simulink model "Samuno_Experimental_2024b"  (R2024b)
settings: Solver=ode4  StartTime=0.0  StopTime=Dur  FixedStep=simulation_ts  RelTol=1e-3  AbsTol=1e-3
InitFcn:
  | run("init_parts.m");
model workspace (MAT data in the model file):
  Control_Range_Lim = 0.2086
  D_Heading = 0
  I_Heading = 0
  P_Heading = 1
  control_ts = 0.4
  kd_pitch = 0
  kd_roll = 0.1
  kp_pitch = 4
  kp_roll = 4
  random_velocity = 0.72
  switch_val = 0.1032
values from neighbouring files (symbols this model uses):
  Force_Scale = 1    [init_parts.m]
  gravity = 9.81    [init_parts.m]
  m = (4*pi*rho*a*b*b)/3    (= 4.90497489324)    [init_parts.m]
  noise_mean = 1    [init_parts.m]
  noise_sample_time = 0.001    [init_parts.m]
  noise_var = 0.001    [init_parts.m]
  Nose = evalin('base', 'Nose')    [createSimulinkGUI_2024b.m]
  xCOB = xSliderCOB.Value    [createSimulinkGUI_2024b.m]    (also in init_parts.m = 0)
  zCOB = ySliderCOB.Value    [createSimulinkGUI_2024b.m]    (also in init_parts.m = 0)
undefined symbols (not defined in the file or in its folder): Caudal, colors, Mid_Body, Mid_Fins, Pect, Pedunc, X, Y, Z
libraries: nesl_utility x92, sm_lib x60
(part 3 of 3)

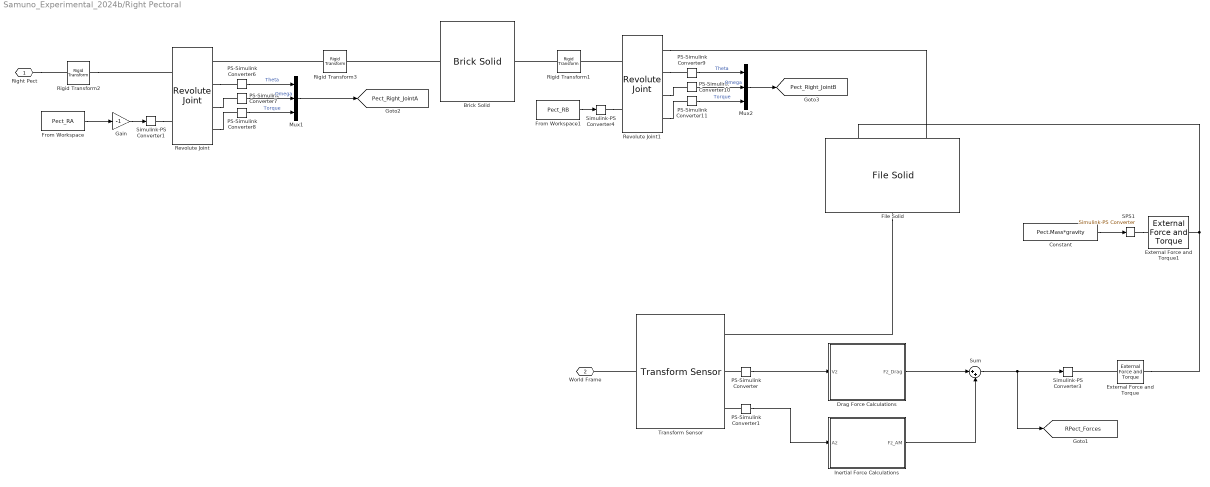
== system Samuno_Experimental_2024b/Right Pectoral ==
  Brick Solid : sm_lib/Body Elements/Brick Solid  BrickDimensions=[.01 .001 .001]  BrickDimensionsUnits=m  ExportEntireGeometry=off  InertiaType=CalculateFromGeometry  BasedOnType=Mass  Density=1000  DensityUnits=kg/m^3  Mass=0  MassUnits=kg  CenterOfMass=[0 0 0]  CenterOfMassUnits=m  MomentsOfInertia=[1 1 1]  MomentsOfInertiaUnits=kg*m^2  ProductsOfInertia=[0 0 0]  ProductsOfInertiaUnits=kg*m^2  GraphicType=FromGeometry  MarkerShape=Sphere  MarkerSize=10  GraphicVisPropType=SimpleVisualProperties  GraphicDiffuseColor=[0.5 0.5 0.5]  GraphicOpacity=1  GraphicSpecularColor=[0.5 0.5 0.5 1.0]  GraphicAmbientColor=[0.15 0.15 0.15 1.0]  GraphicEmissiveColor=[0.0 0.0 0.0 1.0]  GraphicShininess=75  DoExposeReferenceFrame=on  SerializedFrames=<Frames><Frame><Id>Frame1</Id><Value><Name>F1</Name><Origin><Source>ReferenceFrame</Source><FeatureName></FeatureName></Origin><PrimaryAxis><DefinedDirection>+Y</DefinedDirection><Source>GeometricFeature</Source><SourceDirection>+Z</SourceDirection><FeatureName>-y +z curve</FeatureName></PrimaryAxis><SecondaryAxis><DefinedDirection>+X</DefinedDirection><Source>GeometricFeature</Source><SourceDirection>+X</SourceDirection><FeatureName>-z +x curve</FeatureName></SecondaryAxis></Value></Frame></Frames>
  Constant : Constant  Value=Pect.Mass*gravity
  Drag Force Calculations : Subsystem
  External Force and Torque : sm_lib/Forces and Torques/External Force and Torque  EnableForceX=off  EnableForceY=off  EnableForceZ=on  EnableForce=off  ForceResolutionFrame=AttachedFrame  EnableTorqueX=off  EnableTorqueY=off  EnableTorqueZ=off  EnableTorque=off  TorqueResolutionFrame=AttachedFrame
  External Force and Torque1 : sm_lib/Forces and Torques/External Force and Torque  EnableForceX=off  EnableForceY=off  EnableForceZ=on  EnableForce=off  ForceResolutionFrame=World  EnableTorqueX=off  EnableTorqueY=off  EnableTorqueZ=off  EnableTorque=off  TorqueResolutionFrame=AttachedFrame
  File Solid : sm_lib/Body Elements/File Solid  ExtGeomFileName=geometries\webbing_pect.stp  UnitType=FromFile  ExtGeomFileUnits=m  StepReaderType=HEX  ExportConvexHullGeometry=off  InertiaType=Custom  BasedOnType=DensityFromFile  Density=1000  DensityUnits=kg/m^3  Mass=Pect.Mass  MassUnits=kg  CenterOfMass=Pect.CoM  CenterOfMassUnits=m  MomentsOfInertia=Pect.MoI  MomentsOfInertiaUnits=kg*m^2  ProductsOfInertia=Pect.PoI  ProductsOfInertiaUnits=kg*m^2  GraphicType=FromGeometry  MarkerShape=Sphere  MarkerSize=10  GraphicVisPropType=SimpleVisualProperties  GraphicDiffuseColor=colors.pectR  GraphicOpacity=1.0  GraphicSpecularColor=[0.5 0.5 0.5 1.0]  GraphicAmbientColor=[0.15 0.15 0.15 1.0]  GraphicEmissiveColor=[0.0 0.0 0.0 1.0]  GraphicShininess=75  DoExposeReferenceFrame=off  SerializedFrames=<Frames><Frame><Id>Frame2</Id><Value><Name>CoM</Name><Origin><Source>CenterOfMassFrame</Source><FeatureName></FeatureName></Origin><PrimaryAxis><DefinedDirection>+X</DefinedDirection><Source>ReferenceFrame</Source><SourceDirection>+Z</SourceDirection><FeatureName></FeatureName></PrimaryAxis><SecondaryAxis><DefinedDirection>+Z</DefinedDirection><Source>ReferenceFrame</Source><SourceDirection>+X</SourceDirection><FeatureName></FeatureName></SecondaryAxis></Value></Frame><Frame><Id>Frame3</Id><Value><Name>Tip_Offset</Name><Origin><Source>GeometricFeature</Source><FeatureName>segment 12</FeatureName></Origin><PrimaryAxis><DefinedDirection>+X</DefinedDirection><Source>ReferenceFrame</Source><SourceDirection>+Z</SourceDirection><FeatureName></FeatureName></PrimaryAxis><SecondaryAxis><DefinedDirection>+Z</DefinedDirection><Source>ReferenceFrame</Source><SourceDirection>+X</SourceDirection><FeatureName></FeatureName></SecondaryAxis></Value></Frame><Frame><Id>Frame4</Id><Value><Name>Pin2</Name><Origin><Source>ReferenceFrame</Source><FeatureName></FeatureName></Origin><PrimaryAxis><DefinedDirection>+Z</DefinedDirection><Source>ReferenceFrame</Source><SourceDirection>+Z</SourceDirection><FeatureName></FeatureName></PrimaryAxis><SecondaryAxis><DefinedDirection>+Y</DefinedDirection><Source>ReferenceFrame</Source><SourceDirection>+X</SourceDirection><FeatureName></FeatureName></SecondaryAxis></Value></Frame></Frames>
  From Workspace : FromWorkspace  VariableName=Pect_RA
  From Workspace1 : FromWorkspace  VariableName=Pect_RB
  Gain : Gain  Gain=-1
  Inertial Force Calculations : Subsystem
  Mux1 : Mux  Inputs=3
  Mux2 : Mux  Inputs=3
  PS-Simulink Converter{,1,6..11} (8 alike) : nesl_utility/PS-Simulink Converter  PhysicalDomain=network_engine_domain  SubClassName=ps_output  LeftPortType=input  RightPortType=output  PseudoPeriodic=off  Frequencies=[]  VectorFormat=inherit  Unit=inherit  AffineConversion=off
  Revolute Joint : sm_lib/Joints/Revolute Joint  JointMode=Normal  CompositeWrenchDir=FollowerOnBase  CompositeWrenchFrame=BaseFrame  SenseConstraintForce=off  SenseConstraintTorque=off  SenseTotalForce=off  SenseTotalTorque=off  PositionTargetSpecify=off  PositionTargetPriority=High  PositionTargetValue=0  PositionTargetValueUnits=deg  VelocityTargetSpecify=off  VelocityTargetPriority=High  VelocityTargetValue=0  VelocityTargetValueUnits=deg/s  EquilibriumPosition=0  EquilibriumPositionUnits=deg  SpringStiffness=0  SpringStiffnessUnits=N*m/deg  DampingCoefficient=0  DampingCoefficientUnits=N*m/(deg/s)  LowerLimitSpecify=off  LowerLimitBound=-90  LowerLimitBoundUnits=deg  LowerLimitStiffness=1e4  LowerLimitStiffnessUnits=N*m/deg  LowerLimitDamping=10  LowerLimitDampingUnits=N*m/(deg/s)  LowerLimitTransitionRegionWidth=0.1  LowerLimitTransitionRegionWidthUnits=deg  UpperLimitSpecify=off  UpperLimitBound=90  UpperLimitBoundUnits=deg  UpperLimitStiffness=1e4  UpperLimitStiffnessUnits=N*m/deg  UpperLimitDamping=10  UpperLimitDampingUnits=N*m/(deg/s)  UpperLimitTransitionRegionWidth=0.1  UpperLimitTransitionRegionWidthUnits=deg  TorqueActuationMode=ComputedTorque  MotionActuationMode=InputMotion  SensePosition=on  SenseVelocity=on  SenseAcceleration=off  SenseTorqueForce=on  SenseLowerLimitTorqueForce=off  SenseUpperLimitTorqueForce=off
  Revolute Joint1 : sm_lib/Joints/Revolute Joint  JointMode=Normal  CompositeWrenchDir=FollowerOnBase  CompositeWrenchFrame=BaseFrame  SenseConstraintForce=off  SenseConstraintTorque=off  SenseTotalForce=off  SenseTotalTorque=off  PositionTargetSpecify=off  PositionTargetPriority=High  PositionTargetValue=0  PositionTargetValueUnits=deg  VelocityTargetSpecify=off  VelocityTargetPriority=High  VelocityTargetValue=0  VelocityTargetValueUnits=deg/s  EquilibriumPosition=0  EquilibriumPositionUnits=deg  SpringStiffness=0  SpringStiffnessUnits=N*m/deg  DampingCoefficient=0  DampingCoefficientUnits=N*m/(deg/s)  LowerLimitSpecify=off  LowerLimitBound=-90  LowerLimitBoundUnits=deg  LowerLimitStiffness=1e4  LowerLimitStiffnessUnits=N*m/deg  LowerLimitDamping=10  LowerLimitDampingUnits=N*m/(deg/s)  LowerLimitTransitionRegionWidth=0.1  LowerLimitTransitionRegionWidthUnits=deg  UpperLimitSpecify=off  UpperLimitBound=90  UpperLimitBoundUnits=deg  UpperLimitStiffness=1e4  UpperLimitStiffnessUnits=N*m/deg  UpperLimitDamping=10  UpperLimitDampingUnits=N*m/(deg/s)  UpperLimitTransitionRegionWidth=0.1  UpperLimitTransitionRegionWidthUnits=deg  TorqueActuationMode=ComputedTorque  MotionActuationMode=InputMotion  SensePosition=on  SenseVelocity=on  SenseAcceleration=off  SenseTorqueForce=on  SenseLowerLimitTorqueForce=off  SenseUpperLimitTorqueForce=off
  Rigid Transform1 : sm_lib/Frames and Transforms/Rigid Transform  RotationMethod=StandardAxis  FollAlignAxisA=+X  BaseAlignAxisA=+Y  FollAlignAxisB=+Y  BaseAlignAxisB=+Z  RotationStandardAxis=-Y  RotationAngle=90  RotationAngleUnits=deg  RotationArbitraryAxis=[0 0 1]  RotationSequenceAxes=FollowerAxes  RotationSequence=XYX  RotationSequenceAngles=[0 0 0]  RotationSequenceAnglesUnits=deg  RotationMatrix=[1 0 0; 0 1 0; 0 0 1]  Quaternion=[1 0 0 0]  TranslationMethod=StandardAxis  TranslationCartesianOffset=[0 0 0]  TranslationCartesianOffsetUnits=cm  TranslationStandardAxis=+Y  TranslationStandardOffset=0  TranslationStandardOffsetUnits=cm  TranslationROffset=0  TranslationROffsetUnits=m  TranslationThetaOffset=0  TranslationThetaOffsetUnits=deg  TranslationZOffset=0  TranslationZOffsetUnits=m
  Rigid Transform2 : sm_lib/Frames and Transforms/Rigid Transform  RotationMethod=StandardAxis  FollAlignAxisA=+X  BaseAlignAxisA=+Y  FollAlignAxisB=+Y  BaseAlignAxisB=+Z  RotationStandardAxis=-X  RotationAngle=90  RotationAngleUnits=deg  RotationArbitraryAxis=[0 0 1]  RotationSequenceAxes=FollowerAxes  RotationSequence=XYX  RotationSequenceAngles=[0 0 0]  RotationSequenceAnglesUnits=deg  RotationMatrix=[1 0 0; 0 1 0; 0 0 1]  Quaternion=[1 0 0 0]  TranslationMethod=StandardAxis  TranslationCartesianOffset=[0 0 0]  TranslationCartesianOffsetUnits=cm  TranslationStandardAxis=+Y  TranslationStandardOffset=0  TranslationStandardOffsetUnits=cm  TranslationROffset=0  TranslationROffsetUnits=m  TranslationThetaOffset=0  TranslationThetaOffsetUnits=deg  TranslationZOffset=0  TranslationZOffsetUnits=m
  Rigid Transform3 : sm_lib/Frames and Transforms/Rigid Transform  RotationMethod=StandardAxis  FollAlignAxisA=+X  BaseAlignAxisA=+Y  FollAlignAxisB=+Y  BaseAlignAxisB=+Z  RotationStandardAxis=+Z  RotationAngle=90  RotationAngleUnits=deg  RotationArbitraryAxis=[0 0 1]  RotationSequenceAxes=FollowerAxes  RotationSequence=XYX  RotationSequenceAngles=[0 0 0]  RotationSequenceAnglesUnits=deg  RotationMatrix=[1 0 0; 0 1 0; 0 0 1]  Quaternion=[1 0 0 0]  TranslationMethod=StandardAxis  TranslationCartesianOffset=[0 0 0]  TranslationCartesianOffsetUnits=cm  TranslationStandardAxis=+Y  TranslationStandardOffset=0  TranslationStandardOffsetUnits=cm  TranslationROffset=0  TranslationROffsetUnits=m  TranslationThetaOffset=0  TranslationThetaOffsetUnits=deg  TranslationZOffset=0  TranslationZOffsetUnits=m
  SPS1 : nesl_utility/Simulink-PS Converter  PhysicalDomain=network_engine_domain  SubClassName=ps_input  LeftPortType=input  RightPortType=output  PseudoPeriodic=off  Frequencies=[]  NoiseDistribution=none  NoiseParameters=[]  Unit=N  AffineConversion=off  FilteringAndDerivatives=provide  SimscapeFilterOrder=1  InputFilterTimeConstant=0.001  UdotUserProvided=0
  Simulink-PS Converter1 : nesl_utility/Simulink-PS Converter  PhysicalDomain=network_engine_domain  SubClassName=ps_input  LeftPortType=input  RightPortType=output  PseudoPeriodic=off  Frequencies=[]  NoiseDistribution=none  NoiseParameters=[]  Unit=rad  AffineConversion=off  FilteringAndDerivatives=filter  SimscapeFilterOrder=2  InputFilterTimeConstant=0.001  UdotUserProvided=0
  Simulink-PS Converter3 : nesl_utility/Simulink-PS Converter  PhysicalDomain=network_engine_domain  SubClassName=ps_input  LeftPortType=input  RightPortType=output  PseudoPeriodic=off  Frequencies=[]  NoiseDistribution=none  NoiseParameters=[]  Unit=1  AffineConversion=off  FilteringAndDerivatives=filter  SimscapeFilterOrder=2  InputFilterTimeConstant=0.001  UdotUserProvided=0
  Simulink-PS Converter4 : nesl_utility/Simulink-PS Converter  PhysicalDomain=network_engine_domain  SubClassName=ps_input  LeftPortType=input  RightPortType=output  PseudoPeriodic=off  Frequencies=[]  NoiseDistribution=none  NoiseParameters=[]  Unit=rad  AffineConversion=off  FilteringAndDerivatives=filter  SimscapeFilterOrder=2  InputFilterTimeConstant=0.001  UdotUserProvided=0
  Sum : Sum  Inputs=|++
  Transform Sensor : sm_lib/Frames and Transforms/Transform Sensor  MeasurementFrame=NonRotatingFollower  RotationSequence=XYX  SenseAngle=off  SenseAxis=off  SenseQ=off  SenseR=off  SenseRotationSequence=off  SenseOmegaX=off  SenseOmegaY=off  SenseOmegaZ=off  SenseOmega=off  SenseQDot=off  SenseRDot=off  SenseRotationSequenceDot=off  SenseAlphaX=off  SenseAlphaY=off  SenseAlphaZ=off  SenseAlpha=off  SenseQDDot=off  SenseRDDot=off  SenseX=off  SenseY=off  SenseZ=off  SenseXYZ=off  SenseRad=off  SenseAzim=off  SenseDist=off  SenseInc=off  SenseXDot=off  SenseYDot=off  SenseZDot=on  SenseXYZDot=off  SenseRadDot=off  SenseAzimDot=off  SenseDistDot=off  SenseIncDot=off  SenseXDDot=off  SenseYDDot=off  SenseZDDot=on  SenseXYZDDot=off  SenseRadDDot=off  SenseAzimDDot=off  SenseDistDDot=off  SenseIncDDot=off
  Right Pect : PMIOPort  Side=Left
  World Frame : PMIOPort  Port=2  Side=Left
  tag scope: Pect_Right_JointA=global, Pect_Right_JointB=global, RPect_Forces=global
  wires:
  Inertial Force Calculations/1(Fz_AM) -> Sum/2
  Drag Force Calculations/1(Fz_Drag) -> Sum/1
  PS-Simulink Converter/1 -> Drag Force Calculations/1(Vz)
  PS-Simulink Converter1/1 -> Inertial Force Calculations/1(Az)
  Constant/1 -> SPS1/1
  Sum/1 -> [RPect_Forces], Simulink-PS Converter3/1
  Mux1/1 -> [Pect_Right_JointA]
  PS-Simulink Converter6/1 -> Mux1/1  "Theta"
  From Workspace1/1 -> Simulink-PS Converter4/1
  PS-Simulink Converter9/1 -> Mux2/1  "Theta"
  PS-Simulink Converter11/1 -> Mux2/3  "Torque"
  PS-Simulink Converter8/1 -> Mux1/3  "Torque"
  PS-Simulink Converter10/1 -> Mux2/2  "Omega"
  Mux2/1 -> [Pect_Right_JointB]
  PS-Simulink Converter7/1 -> Mux1/2  "Omega"
  From Workspace/1 -> Gain/1
  Gain/1 -> Simulink-PS Converter1/1
  connections:
  External Force and Torque/RConn1 -- File Solid/LConn1 -- External Force and Torque1/RConn1
  Transform Sensor/LConn1 -- World Frame/RConn1
  PS-Simulink Converter1/LConn1 -- Transform Sensor/RConn3
  PS-Simulink Converter/LConn1 -- Transform Sensor/RConn2
  External Force and Torque/LConn1 -- Simulink-PS Converter3/RConn1
  File Solid/RConn1 -- Transform Sensor/RConn1
  SPS1/RConn1 -- External Force and Torque1/LConn1
  Simulink-PS Converter1/RConn1 -- Revolute Joint/LConn2
  Revolute Joint1/RConn4 -- PS-Simulink Converter11/LConn1
  Revolute Joint1/RConn1 -- File Solid/LConn2
  Rigid Transform1/RConn1 -- Brick Solid/RConn1
  Simulink-PS Converter4/RConn1 -- Revolute Joint1/LConn2
  Revolute Joint/RConn4 -- PS-Simulink Converter8/LConn1
  Revolute Joint/RConn3 -- PS-Simulink Converter7/LConn1
  Revolute Joint1/RConn2 -- PS-Simulink Converter9/LConn1
  Revolute Joint/RConn2 -- PS-Simulink Converter6/LConn1
  Rigid Transform3/RConn1 -- Revolute Joint/RConn1
  Right Pect/RConn1 -- Rigid Transform2/RConn1
  Revolute Joint1/RConn3 -- PS-Simulink Converter10/LConn1
  Rigid Transform2/LConn1 -- Revolute Joint/LConn1
  Revolute Joint1/LConn1 -- Rigid Transform1/LConn1
  Brick Solid/LConn1 -- Rigid Transform3/LConn1

== system Samuno_Experimental_2024b/Body - Middle/Drag Force Calculations ==
  vx : Inport
  vy : Inport  Port=2
  vz : Inport  Port=3
  Constant : Constant  Value=-1
  Constant1 : Constant  Value=997
  Constant10 : Constant  Value=Mid_Body.X_Cd
  Constant11 : Constant  Value=Mid_Body.X_Area
  Constant2 : Constant  Value=-1
  Constant3 : Constant  Value=Mid_Body.Y_Cd
  Constant4 : Constant  Value=Mid_Body.Y_Area
  Constant5 : Constant  Value=997
  Constant6 : Constant  Value=Mid_Body.Z_Cd
  Constant7 : Constant  Value=Mid_Body.Z_Area
  Constant8 : Constant  Value=-1
  Constant9 : Constant  Value=997
  MATLAB Function1 : MATLAB Function  TreatAsAtomicUnit=on
  MATLAB Function2 : MATLAB Function  TreatAsAtomicUnit=on
  MATLAB Function3 : MATLAB Function  TreatAsAtomicUnit=on
  Fx_Drag : Outport
  Fy_Drag : Outport  Port=2
  Fz_Drag : Outport  Port=3
  wires:
  vy/1 -> MATLAB Function1/1(vel)
  Constant1/1 -> MATLAB Function1/3(Rho)
  Constant3/1 -> MATLAB Function1/2(Cd)
  Constant/1 -> MATLAB Function1/5(scale)
  MATLAB Function1/1(drag_force) -> Fy_Drag/1
  Constant4/1 -> MATLAB Function1/4(Area)
  Constant5/1 -> MATLAB Function2/3(Rho)
  MATLAB Function2/1(drag_force) -> Fz_Drag/1
  Constant7/1 -> MATLAB Function2/4(Area)
  Constant2/1 -> MATLAB Function2/5(scale)
  vz/1 -> MATLAB Function2/1(vel)
  Constant6/1 -> MATLAB Function2/2(Cd)
  Constant9/1 -> MATLAB Function3/3(Rho)
  MATLAB Function3/1(drag_force) -> Fx_Drag/1
  Constant11/1 -> MATLAB Function3/4(Area)
  Constant8/1 -> MATLAB Function3/5(scale)
  vx/1 -> MATLAB Function3/1(vel)
  Constant10/1 -> MATLAB Function3/2(Cd)

== system Samuno_Experimental_2024b/Body - Middle/Inertial Force Calculations ==
  Ax : Inport
  Ay : Inport  Port=2
  Az : Inport  Port=3
  Constant : Constant  Value=-1
  Constant1 : Constant  Value=-1
  Constant2 : Constant  Value=Mid_Body.X_am
  Constant3 : Constant  Value=Mid_Body.Y_am
  Constant4 : Constant  Value=-1
  Constant5 : Constant  Value=Mid_Body.Z_am
  MATLAB Function1 : MATLAB Function  TreatAsAtomicUnit=on
  MATLAB Function2 : MATLAB Function  TreatAsAtomicUnit=on
  MATLAB Function3 : MATLAB Function  TreatAsAtomicUnit=on
  Transfer Fcn1 : TransferFcn  Numerator=1.5  Denominator=[0.005 1]
  Transfer Fcn2 : TransferFcn  Numerator=1.5  Denominator=[0.005 1]
  Transfer Fcn3 : TransferFcn  Numerator=1.5  Denominator=[0.005 1]
  Fx_AM : Outport
  Fy_AM : Outport  Port=2
  Fz_AM : Outport  Port=3
  wires:
  Constant3/1 -> MATLAB Function1/2(Coeff)
  MATLAB Function1/1(Inertial_Force) -> Transfer Fcn2/1
  Ay/1 -> MATLAB Function1/1(acc)
  Transfer Fcn2/1 -> Fy_AM/1
  Constant/1 -> MATLAB Function1/3(scale)
  MATLAB Function2/1(Inertial_Force) -> Transfer Fcn1/1
  Constant2/1 -> MATLAB Function2/2(Coeff)
  Transfer Fcn1/1 -> Fx_AM/1
  Ax/1 -> MATLAB Function2/1(acc)
  Constant1/1 -> MATLAB Function2/3(scale)
  MATLAB Function3/1(Inertial_Force) -> Transfer Fcn3/1
  Constant5/1 -> MATLAB Function3/2(Coeff)
  Transfer Fcn3/1 -> Fz_AM/1
  Az/1 -> MATLAB Function3/1(acc)
  Constant4/1 -> MATLAB Function3/3(scale)

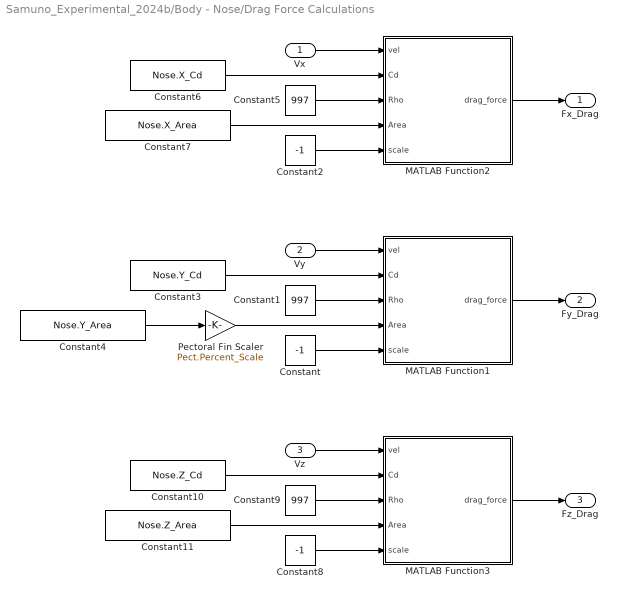
== system Samuno_Experimental_2024b/Body - Nose/Drag Force Calculations ==
  Vx : Inport
  Vy : Inport  Port=2
  Vz : Inport  Port=3
  Constant : Constant  Value=-1
  Constant1 : Constant  Value=997
  Constant10 : Constant  Value=Nose.Z_Cd
  Constant11 : Constant  Value=Nose.Z_Area
  Constant2 : Constant  Value=-1
  Constant3 : Constant  Value=Nose.Y_Cd
  Constant4 : Constant  Value=Nose.Y_Area
  Constant5 : Constant  Value=997
  Constant6 : Constant  Value=Nose.X_Cd
  Constant7 : Constant  Value=Nose.X_Area
  Constant8 : Constant  Value=-1
  Constant9 : Constant  Value=997
  MATLAB Function1 : MATLAB Function  TreatAsAtomicUnit=on
  MATLAB Function2 : MATLAB Function  TreatAsAtomicUnit=on
  MATLAB Function3 : MATLAB Function  TreatAsAtomicUnit=on
  Pectoral Fin Scaler : Gain  Gain=Pect.Percent_Scale
  Fx_Drag : Outport
  Fy_Drag : Outport  Port=2
  Fz_Drag : Outport  Port=3
  wires:
  Constant1/1 -> MATLAB Function1/3(Rho)
  MATLAB Function1/1(drag_force) -> Fy_Drag/1
  Constant4/1 -> Pectoral Fin Scaler/1
  Constant/1 -> MATLAB Function1/5(scale)
  Vy/1 -> MATLAB Function1/1(vel)
  Constant3/1 -> MATLAB Function1/2(Cd)
  Constant6/1 -> MATLAB Function2/2(Cd)
  Constant2/1 -> MATLAB Function2/5(scale)
  Constant7/1 -> MATLAB Function2/4(Area)
  Vx/1 -> MATLAB Function2/1(vel)
  MATLAB Function2/1(drag_force) -> Fx_Drag/1
  Constant5/1 -> MATLAB Function2/3(Rho)
  MATLAB Function3/1(drag_force) -> Fz_Drag/1
  Constant8/1 -> MATLAB Function3/5(scale)
  Constant11/1 -> MATLAB Function3/4(Area)
  Constant10/1 -> MATLAB Function3/2(Cd)
  Vz/1 -> MATLAB Function3/1(vel)
  Constant9/1 -> MATLAB Function3/3(Rho)
  Pectoral Fin Scaler/1 -> MATLAB Function1/4(Area)

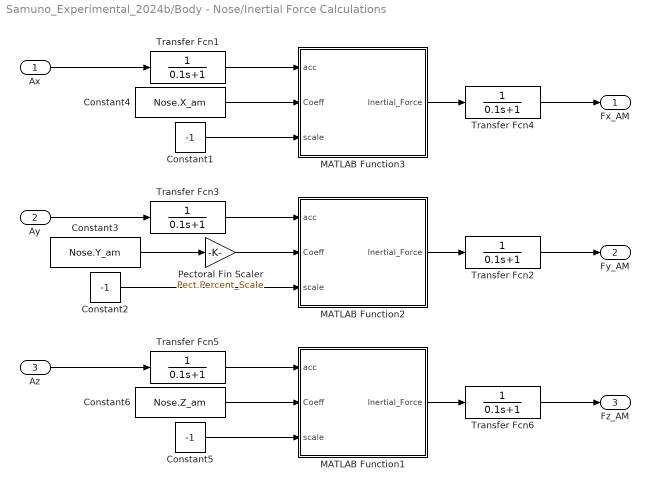
== system Samuno_Experimental_2024b/Body - Nose/Inertial Force Calculations ==
  Ax : Inport
  Ay : Inport  Port=2
  Az : Inport  Port=3
  Constant1 : Constant  Value=-1
  Constant2 : Constant  Value=-1
  Constant3 : Constant  Value=Nose.Y_am
  Constant4 : Constant  Value=Nose.X_am
  Constant5 : Constant  Value=-1
  Constant6 : Constant  Value=Nose.Z_am
  MATLAB Function1 : MATLAB Function  TreatAsAtomicUnit=on
  MATLAB Function2 : MATLAB Function  TreatAsAtomicUnit=on
  MATLAB Function3 : MATLAB Function  TreatAsAtomicUnit=on
  Pectoral Fin Scaler : Gain  Gain=Pect.Percent_Scale
  Transfer Fcn{1..6} (6 alike) : TransferFcn  Denominator=[0.1 1]
  Fx_AM : Outport
  Fy_AM : Outport  Port=2
  Fz_AM : Outport  Port=3
  wires:
  Ax/1 -> Transfer Fcn1/1
  Constant1/1 -> MATLAB Function3/3(scale)
  Transfer Fcn1/1 -> MATLAB Function3/1(acc)
  Constant4/1 -> MATLAB Function3/2(Coeff)
  Transfer Fcn4/1 -> Fx_AM/1
  MATLAB Function3/1(Inertial_Force) -> Transfer Fcn4/1
  Ay/1 -> Transfer Fcn3/1
  Constant2/1 -> MATLAB Function2/3(scale)
  Transfer Fcn3/1 -> MATLAB Function2/1(acc)
  Constant3/1 -> Pectoral Fin Scaler/1
  Transfer Fcn2/1 -> Fy_AM/1
  MATLAB Function2/1(Inertial_Force) -> Transfer Fcn2/1
  Az/1 -> Transfer Fcn5/1
  Constant5/1 -> MATLAB Function1/3(scale)
  Transfer Fcn5/1 -> MATLAB Function1/1(acc)
  Constant6/1 -> MATLAB Function1/2(Coeff)
  Transfer Fcn6/1 -> Fz_AM/1
  MATLAB Function1/1(Inertial_Force) -> Transfer Fcn6/1
  Pectoral Fin Scaler/1 -> MATLAB Function2/2(Coeff)

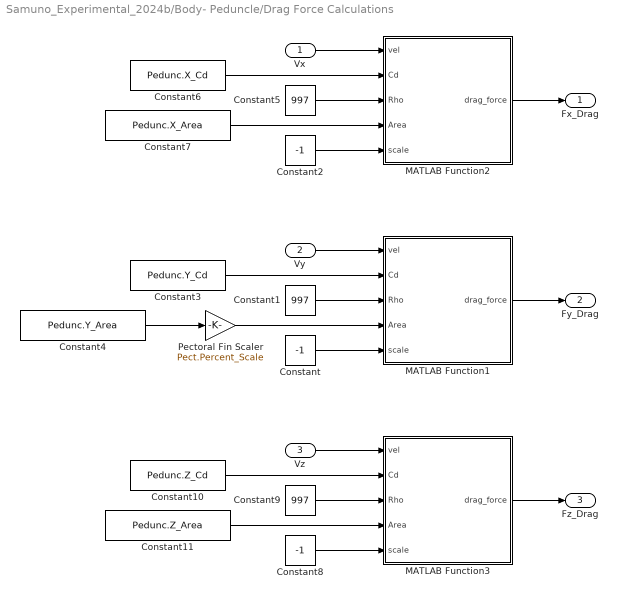
== system Samuno_Experimental_2024b/Body- Peduncle/Drag Force Calculations ==
  Vx : Inport
  Vy : Inport  Port=2
  Vz : Inport  Port=3
  Constant : Constant  Value=-1
  Constant1 : Constant  Value=997
  Constant10 : Constant  Value=Pedunc.Z_Cd
  Constant11 : Constant  Value=Pedunc.Z_Area
  Constant2 : Constant  Value=-1
  Constant3 : Constant  Value=Pedunc.Y_Cd
  Constant4 : Constant  Value=Pedunc.Y_Area
  Constant5 : Constant  Value=997
  Constant6 : Constant  Value=Pedunc.X_Cd
  Constant7 : Constant  Value=Pedunc.X_Area
  Constant8 : Constant  Value=-1
  Constant9 : Constant  Value=997
  MATLAB Function1 : MATLAB Function  TreatAsAtomicUnit=on
  MATLAB Function2 : MATLAB Function  TreatAsAtomicUnit=on
  MATLAB Function3 : MATLAB Function  TreatAsAtomicUnit=on
  Pectoral Fin Scaler : Gain  Gain=Pect.Percent_Scale
  Fx_Drag : Outport
  Fy_Drag : Outport  Port=2
  Fz_Drag : Outport  Port=3
  wires:
  Constant1/1 -> MATLAB Function1/3(Rho)
  MATLAB Function1/1(drag_force) -> Fy_Drag/1
  Constant4/1 -> Pectoral Fin Scaler/1
  Constant/1 -> MATLAB Function1/5(scale)
  Vy/1 -> MATLAB Function1/1(vel)
  Constant3/1 -> MATLAB Function1/2(Cd)
  Constant6/1 -> MATLAB Function2/2(Cd)
  Constant2/1 -> MATLAB Function2/5(scale)
  Constant7/1 -> MATLAB Function2/4(Area)
  Vx/1 -> MATLAB Function2/1(vel)
  MATLAB Function2/1(drag_force) -> Fx_Drag/1
  Constant5/1 -> MATLAB Function2/3(Rho)
  MATLAB Function3/1(drag_force) -> Fz_Drag/1
  Constant8/1 -> MATLAB Function3/5(scale)
  Constant11/1 -> MATLAB Function3/4(Area)
  Constant10/1 -> MATLAB Function3/2(Cd)
  Vz/1 -> MATLAB Function3/1(vel)
  Constant9/1 -> MATLAB Function3/3(Rho)
  Pectoral Fin Scaler/1 -> MATLAB Function1/4(Area)

== system Samuno_Experimental_2024b/Body- Peduncle/Inertial Force Calculations ==
  Ax : Inport
  Ay : Inport  Port=2
  Az : Inport  Port=3
  Constant1 : Constant  Value=-1
  Constant2 : Constant  Value=-1
  Constant3 : Constant  Value=Pedunc.Y_am
  Constant4 : Constant  Value=Pedunc.X_am
  Constant5 : Constant  Value=-1
  Constant6 : Constant  Value=Pedunc.Z_am
  MATLAB Function1 : MATLAB Function  TreatAsAtomicUnit=on
  MATLAB Function2 : MATLAB Function  TreatAsAtomicUnit=on
  MATLAB Function3 : MATLAB Function  TreatAsAtomicUnit=on
  Pectoral Fin Scaler : Gain  Gain=Pect.Percent_Scale
  Transfer Fcn1 : TransferFcn  Numerator=1.5  Denominator=[0.005 1]
  Transfer Fcn2 : TransferFcn  Numerator=1.5  Denominator=[0.005 1]
  Transfer Fcn3 : TransferFcn  Numerator=1.5  Denominator=[0.005 1]
  Fx_AM : Outport
  Fy_AM : Outport  Port=2
  Fz_AM : Outport  Port=3
  wires:
  Constant1/1 -> MATLAB Function3/3(scale)
  Ax/1 -> MATLAB Function3/1(acc)
  Constant4/1 -> MATLAB Function3/2(Coeff)
  Transfer Fcn1/1 -> Fx_AM/1
  MATLAB Function3/1(Inertial_Force) -> Transfer Fcn1/1
  Constant2/1 -> MATLAB Function2/3(scale)
  Ay/1 -> MATLAB Function2/1(acc)
  Constant3/1 -> Pectoral Fin Scaler/1
  Transfer Fcn2/1 -> Fy_AM/1
  MATLAB Function2/1(Inertial_Force) -> Transfer Fcn2/1
  Constant5/1 -> MATLAB Function1/3(scale)
  Az/1 -> MATLAB Function1/1(acc)
  Constant6/1 -> MATLAB Function1/2(Coeff)
  Transfer Fcn3/1 -> Fz_AM/1
  MATLAB Function1/1(Inertial_Force) -> Transfer Fcn3/1
  Pectoral Fin Scaler/1 -> MATLAB Function2/2(Coeff)

== system Samuno_Experimental_2024b/Caudal Fin/Drag Force Calculations ==
  vy : Inport
  Constant3 : Constant  Value=Caudal.Y_Area
  Constant5 : Constant  Value=-1
  Constant6 : Constant  Value=997
  Constant8 : Constant  Value=Caudal.Y_Cd
  MATLAB Function1 : MATLAB Function  TreatAsAtomicUnit=on
  Fy_Drag : Outport
  wires:
  MATLAB Function1/1(drag_force) -> Fy_Drag/1
  vy/1 -> MATLAB Function1/1(vel)
  Constant3/1 -> MATLAB Function1/4(Area)
  Constant6/1 -> MATLAB Function1/3(Rho)
  Constant8/1 -> MATLAB Function1/2(Cd)
  Constant5/1 -> MATLAB Function1/5(scale)

== system Samuno_Experimental_2024b/Caudal Fin/Inertial Force Calculations ==
  Ay : Inport
  Constant : Constant  Value=-1
  Constant3 : Constant  Value=Caudal.Y_am
  MATLAB Function1 : MATLAB Function  TreatAsAtomicUnit=on
  Transfer Fcn1 : TransferFcn  Numerator=1.5  Denominator=[0.005 1]
  Fy_AM : Outport
  wires:
  Constant3/1 -> MATLAB Function1/2(Coeff)
  MATLAB Function1/1(Inertial_Force) -> Transfer Fcn1/1
  Transfer Fcn1/1 -> Fy_AM/1
  Constant/1 -> MATLAB Function1/3(scale)
  Ay/1 -> MATLAB Function1/1(acc)

== system Samuno_Experimental_2024b/Dorsal-Anal Fins/Drag Force Calculations ==
  vy : Inport
  Constant3 : Constant  Value=Mid_Fins.Y_Cd
  Constant4 : Constant  Value=Mid_Fins.Y_Area
  Constant8 : Constant  Value=-1
  Constant9 : Constant  Value=997
  MATLAB Function1 : MATLAB Function  TreatAsAtomicUnit=on
  Fy_Drag : Outport
  wires:
  MATLAB Function1/1(drag_force) -> Fy_Drag/1
  Constant8/1 -> MATLAB Function1/5(scale)
  Constant9/1 -> MATLAB Function1/3(Rho)
  Constant4/1 -> MATLAB Function1/4(Area)
  Constant3/1 -> MATLAB Function1/2(Cd)
  vy/1 -> MATLAB Function1/1(vel)

== system Samuno_Experimental_2024b/Dorsal-Anal Fins/Drag Force Calculations1 ==
  vy : Inport
  Constant1 : Constant  Value=Mid_Fins.Y_Cd
  Constant3 : Constant  Value=997
  Constant4 : Constant  Value=Mid_Fins.Y_Area
  Constant8 : Constant  Value=-1
  MATLAB Function1 : MATLAB Function  TreatAsAtomicUnit=on
  Fy_Drag : Outport
  wires:
  vy/1 -> MATLAB Function1/1(vel)
  Constant4/1 -> MATLAB Function1/4(Area)
  MATLAB Function1/1(drag_force) -> Fy_Drag/1
  Constant1/1 -> MATLAB Function1/2(Cd)
  Constant3/1 -> MATLAB Function1/3(Rho)
  Constant8/1 -> MATLAB Function1/5(scale)

== system Samuno_Experimental_2024b/Dorsal-Anal Fins/Inertial Force Calculations ==
  Ay : Inport
  Constant : Constant  Value=-1
  Constant3 : Constant  Value=Mid_Fins.Y_am
  MATLAB Function1 : MATLAB Function  TreatAsAtomicUnit=on
  Transfer Fcn1 : TransferFcn  Numerator=1.5  Denominator=[0.005 1]
  Fy_AM : Outport
  wires:
  Constant3/1 -> MATLAB Function1/2(Coeff)
  MATLAB Function1/1(Inertial_Force) -> Transfer Fcn1/1
  Ay/1 -> MATLAB Function1/1(acc)
  Constant/1 -> MATLAB Function1/3(scale)
  Transfer Fcn1/1 -> Fy_AM/1

== system Samuno_Experimental_2024b/Dorsal-Anal Fins/Inertial Force Calculations1 ==
  Ay1 : Inport
  Constant : Constant  Value=-1
  Constant1 : Constant  Value=Mid_Fins.Y_am
  MATLAB Function2 : MATLAB Function  TreatAsAtomicUnit=on
  Transfer Fcn2 : TransferFcn  Numerator=1.5  Denominator=[0.005 1]
  Fy_AM1 : Outport
  wires:
  Transfer Fcn2/1 -> Fy_AM1/1
  Constant/1 -> MATLAB Function2/3(scale)
  MATLAB Function2/1(Inertial_Force) -> Transfer Fcn2/1
  Ay1/1 -> MATLAB Function2/1(acc)
  Constant1/1 -> MATLAB Function2/2(Coeff)

== system Samuno_Experimental_2024b/Left Pectoral/Drag Force Calculations ==
  Vz : Inport
  Constant1 : Constant  Value=Pect.Y_Cd
  Constant3 : Constant  Value=997
  Constant4 : Constant  Value=Pect.Y_Area
  Constant8 : Constant  Value=-1
  MATLAB Function1 : MATLAB Function  TreatAsAtomicUnit=on
  Fz_Drag : Outport
  wires:
  Constant1/1 -> MATLAB Function1/2(Cd)
  Constant3/1 -> MATLAB Function1/3(Rho)
  Constant8/1 -> MATLAB Function1/5(scale)
  Constant4/1 -> MATLAB Function1/4(Area)
  MATLAB Function1/1(drag_force) -> Fz_Drag/1
  Vz/1 -> MATLAB Function1/1(vel)

== system Samuno_Experimental_2024b/Left Pectoral/Inertial Force Calculations ==
  Az : Inport
  Constant : Constant  Value=-1
  Constant1 : Constant  Value=Pect.Y_am
  MATLAB Function2 : MATLAB Function  TreatAsAtomicUnit=on
  Transfer Fcn1 : TransferFcn  Denominator=[0.1 1]
  Transfer Fcn3 : TransferFcn  Denominator=[0.1 1]
  Fz_AM : Outport
  wires:
  MATLAB Function2/1(Inertial_Force) -> Transfer Fcn1/1
  Transfer Fcn1/1 -> Fz_AM/1
  Az/1 -> Transfer Fcn3/1
  Constant1/1 -> MATLAB Function2/2(Coeff)
  Transfer Fcn3/1 -> MATLAB Function2/1(acc)
  Constant/1 -> MATLAB Function2/3(scale)

== system Samuno_Experimental_2024b/Right Pectoral/Drag Force Calculations ==
  Vz : Inport
  Constant1 : Constant  Value=Pect.Y_Cd
  Constant3 : Constant  Value=997
  Constant4 : Constant  Value=Pect.Y_Area
  Constant8 : Constant  Value=-1
  MATLAB Function1 : MATLAB Function  TreatAsAtomicUnit=on
  Fz_Drag : Outport
  wires:
  Constant1/1 -> MATLAB Function1/2(Cd)
  Constant3/1 -> MATLAB Function1/3(Rho)
  Constant8/1 -> MATLAB Function1/5(scale)
  Constant4/1 -> MATLAB Function1/4(Area)
  MATLAB Function1/1(drag_force) -> Fz_Drag/1
  Vz/1 -> MATLAB Function1/1(vel)

== system Samuno_Experimental_2024b/Right Pectoral/Inertial Force Calculations ==
  Az : Inport
  Constant : Constant  Value=-1
  Constant1 : Constant  Value=Pect.Y_am
  MATLAB Function2 : MATLAB Function  TreatAsAtomicUnit=on
  Transfer Fcn1 : TransferFcn  Numerator=1.5  Denominator=[0.005 1]
  Fz_AM : Outport
  wires:
  MATLAB Function2/1(Inertial_Force) -> Transfer Fcn1/1
  Transfer Fcn1/1 -> Fz_AM/1
  Constant1/1 -> MATLAB Function2/2(Coeff)
  Az/1 -> MATLAB Function2/1(acc)
  Constant/1 -> MATLAB Function2/3(scale)

== matlab function Samuno_Experimental_2024b/Body - Middle/Drag Force Calculations/MATLAB Function3 ==
  data: vel input; drag_force output; Cd input; Rho input; Area input; scale input
function drag_force=Drag_Force(vel,Cd,Rho,Area,scale)

    drag_force=(1/2)*Rho*Cd*(Area)*(abs(vel)*vel)*scale;

end

== matlab function Samuno_Experimental_2024b/Calculate MoI/MATLAB Function ==
  data: matrix input; main_diag output
function main_diag = getDiagonals(matrix)
    % Check if the input is a 3x3 matrix
    if size(matrix, 1) ~= 3 || size(matrix, 2) ~= 3
        error('Input must be a 3x3 matrix');
    end

    % Extract the main diagonal
    main_diag = diag(matrix);
    
end

== matlab function Samuno_Experimental_2024b/Body - Middle/Inertial Force Calculations/MATLAB Function1 ==
  data: acc input; Inertial_Force output; Coeff input; scale input
function Inertial_Force=Added_Mass(acc,Coeff,scale)

    Inertial_Force=scale*acc*Coeff;

end

== matlab function Samuno_Experimental_2024b/Caudal Fin/Drag Force Calculations/MATLAB Function1 ==
  data: vel input; drag_force output; Cd input; Rho input; Area input; scale input
function drag_force=Drag_Force(vel,Cd,Rho,Area,scale)

    drag_force=(1/2)*Rho*Cd*(Area)*(abs(vel)*vel)*scale;

end

== matlab function Samuno_Experimental_2024b/Body - Middle/Inertial Force Calculations/MATLAB Function2 ==
  data: acc input; Inertial_Force output; Coeff input; scale input
function Inertial_Force=Added_Mass(acc,Coeff,scale)

    Inertial_Force=scale*acc*Coeff;

end

== matlab function Samuno_Experimental_2024b/Body - Middle/Inertial Force Calculations/MATLAB Function3 ==
  data: acc input; Inertial_Force output; Coeff input; scale input
function Inertial_Force=Added_Mass(acc,Coeff,scale)

    Inertial_Force=scale*acc*Coeff;

end

== matlab function Samuno_Experimental_2024b/Body - Nose/Drag Force Calculations/MATLAB Function2 ==
  data: vel input; drag_force output; Cd input; Rho input; Area input; scale input
function drag_force=Drag_Force(vel,Cd,Rho,Area,scale)

    drag_force=(1/2)*Rho*Cd*(Area)*(abs(vel)*vel)*scale;

end

== matlab function Samuno_Experimental_2024b/Body - Nose/Drag Force Calculations/MATLAB Function3 ==
  data: vel input; drag_force output; Cd input; Rho input; Area input; scale input
function drag_force=Drag_Force(vel,Cd,Rho,Area,scale)

    drag_force=(1/2)*Rho*Cd*(Area)*(abs(vel)*vel)*scale;

end

== matlab function Samuno_Experimental_2024b/Body - Nose/Inertial Force Calculations/MATLAB Function3 ==
  data: acc input; Inertial_Force output; Coeff input; scale input
function Inertial_Force=Added_Mass(acc,Coeff,scale)

    Inertial_Force=scale*acc*Coeff;

end

== matlab function Samuno_Experimental_2024b/Right Pectoral/Drag Force Calculations/MATLAB Function1 ==
  data: vel input; drag_force output; Cd input; Rho input; Area input; scale input
function drag_force=Drag_Force(vel,Cd,Rho,Area,scale)

    drag_force=(1/2)*Rho*Cd*(Area)*(abs(vel)*vel)*scale;

end

== matlab function Samuno_Experimental_2024b/Body- Peduncle/Drag Force Calculations/MATLAB Function3 ==
  data: vel input; drag_force output; Cd input; Rho input; Area input; scale input
function drag_force=Drag_Force(vel,Cd,Rho,Area,scale)

    drag_force=(1/2)*Rho*Cd*(Area)*(abs(vel)*vel)*scale;

end

== matlab function Samuno_Experimental_2024b/Body - Nose/Inertial Force Calculations/MATLAB Function2 ==
  data: acc input; Inertial_Force output; Coeff input; scale input
function Inertial_Force=Added_Mass(acc,Coeff,scale)

    Inertial_Force=scale*acc*Coeff;

end

== matlab function Samuno_Experimental_2024b/Body - Nose/Inertial Force Calculations/MATLAB Function1 ==
  data: acc input; Inertial_Force output; Coeff input; scale input
function Inertial_Force=Added_Mass(acc,Coeff,scale)

    Inertial_Force=scale*(acc)*Coeff;

end

== matlab function Samuno_Experimental_2024b/Dorsal-Anal Fins/Drag Force Calculations1/MATLAB Function1 ==
  data: vel input; drag_force output; Cd input; Rho input; Area input; scale input
function drag_force=Drag_Force(vel,Cd,Rho,Area,scale)

    drag_force=(1/2)*Rho*Cd*(Area)*(abs(vel)*vel)*scale;

end

== matlab function Samuno_Experimental_2024b/Left Pectoral/Drag Force Calculations/MATLAB Function1 ==
  data: vel input; drag_force output; Cd input; Rho input; Area input; scale input
function drag_force=Drag_Force(vel,Cd,Rho,Area,scale)

    drag_force=(1/2)*Rho*Cd*(Area)*(abs(vel)*vel)*scale;

end

== matlab function Samuno_Experimental_2024b/Left Pectoral/Inertial Force Calculations/MATLAB Function2 ==
  data: acc input; Inertial_Force output; Coeff input; scale input
function Inertial_Force=Added_Mass(acc,Coeff,scale)

    Inertial_Force=scale*acc*Coeff;

end

== matlab function Samuno_Experimental_2024b/Body- Peduncle/Inertial Force Calculations/MATLAB Function1 ==
  data: acc input; Inertial_Force output; Coeff input; scale input
function Inertial_Force=Added_Mass(acc,Coeff,scale)

    Inertial_Force=scale*(acc)*Coeff;

end

== matlab function Samuno_Experimental_2024b/Body- Peduncle/Inertial Force Calculations/MATLAB Function2 ==
  data: acc input; Inertial_Force output; Coeff input; scale input
function Inertial_Force=Added_Mass(acc,Coeff,scale)

    Inertial_Force=scale*acc*Coeff;

end

== matlab function Samuno_Experimental_2024b/Body- Peduncle/Inertial Force Calculations/MATLAB Function3 ==
  data: acc input; Inertial_Force output; Coeff input; scale input
function Inertial_Force=Added_Mass(acc,Coeff,scale)

    Inertial_Force=scale*acc*Coeff;

end

== matlab function Samuno_Experimental_2024b/Right Pectoral/Inertial Force Calculations/MATLAB Function2 ==
  data: acc input; Inertial_Force output; Coeff input; scale input
function Inertial_Force=Added_Mass(acc,Coeff,scale)

    Inertial_Force=scale*acc*Coeff;

end

== matlab function Samuno_Experimental_2024b/Dorsal-Anal Fins/Inertial Force Calculations/MATLAB Function1 ==
  data: acc input; Inertial_Force output; Coeff input; scale input
function Inertial_Force=Added_Mass(acc,Coeff,scale)

    Inertial_Force=scale*acc*Coeff;

end

== matlab function Samuno_Experimental_2024b/Caudal Fin/Inertial Force Calculations/MATLAB Function1 ==
  data: acc input; Inertial_Force output; Coeff input; scale input
function Inertial_Force=Added_Mass(acc,Coeff,scale)

    Inertial_Force=scale*acc*Coeff;

end

== matlab function Samuno_Experimental_2024b/Body- Peduncle/Drag Force Calculations/MATLAB Function1 ==
  data: vel input; drag_force output; Cd input; Rho input; Area input; scale input
function drag_force=Drag_Force(vel,Cd,Rho,Area,scale)

    drag_force=(1/2)*Rho*Cd*(Area)*(abs(vel)*vel)*scale;

end

== matlab function Samuno_Experimental_2024b/Body- Peduncle/Drag Force Calculations/MATLAB Function2 ==
  data: vel input; drag_force output; Cd input; Rho input; Area input; scale input
function drag_force=Drag_Force(vel,Cd,Rho,Area,scale)

    drag_force=(1/2)*Rho*Cd*(Area)*(abs(vel)*vel)*scale;

end

== matlab function Samuno_Experimental_2024b/Body - Middle/Drag Force Calculations/MATLAB Function1 ==
  data: vel input; drag_force output; Cd input; Rho input; Area input; scale input
function drag_force=Drag_Force(vel,Cd,Rho,Area,scale)

    drag_force=(1/2)*Rho*Cd*(Area)*(abs(vel)*vel)*scale;

end

== matlab function Samuno_Experimental_2024b/Body - Middle/Drag Force Calculations/MATLAB Function2 ==
  data: vel input; drag_force output; Cd input; Rho input; Area input; scale input
function drag_force=Drag_Force(vel,Cd,Rho,Area,scale)

    drag_force=(1/2)*Rho*Cd*(Area)*(abs(vel)*vel)*scale;

end

== matlab function Samuno_Experimental_2024b/Body - Nose/Drag Force Calculations/MATLAB Function1 ==
  data: vel input; drag_force output; Cd input; Rho input; Area input; scale input
function drag_force=Drag_Force(vel,Cd,Rho,Area,scale)

    drag_force=(1/2)*Rho*Cd*(Area)*(abs(vel)*vel)*scale;

end

== matlab function Samuno_Experimental_2024b/Dorsal-Anal Fins/Inertial Force Calculations1/MATLAB Function2 ==
  data: acc input; Inertial_Force output; Coeff input; scale input
function Inertial_Force=Added_Mass(acc,Coeff,scale)

    Inertial_Force=scale*acc*Coeff;

end

== matlab function Samuno_Experimental_2024b/Dorsal-Anal Fins/Drag Force Calculations/MATLAB Function1 ==
  data: vel input; drag_force output; Cd input; Rho input; Area input; scale input
function drag_force=Drag_Force(vel,Cd,Rho,Area,scale)

    drag_force=(1/2)*Rho*Cd*(Area)*(abs(vel)*vel)*scale;

end
